simulink model "multi_model_sim_with_switching"  (R2013b)
settings: Solver=ode45  StartTime=0.0  StopTime=20  RelTol=1e-3
values from neighbouring files (symbols this model uses):
  C1d = [1 0]    [multi_model_sim_init.m]
  C1n = [C.Kp C.Ki]    [multi_model_sim_init.m]
  C2d = [1 0]    [multi_model_sim_init.m]
  C2n = [C.Kp C.Ki]    [multi_model_sim_init.m]
  C3d = [1 0]    [multi_model_sim_init.m]
  C3n = [C.Kp C.Ki]    [multi_model_sim_init.m]
  error_gain = 2    [multi_model_sim_init.m]
  P1d = [0.9125 1]    [multi_model_sim_init.m]
  P1n = [3.7]    [multi_model_sim_init.m]
  P2d = [1.075 1]    [multi_model_sim_init.m]
  P2n = [4]    [multi_model_sim_init.m]
  P3d = [0.7875 1]    [multi_model_sim_init.m]
  P3n = [1.78]    [multi_model_sim_init.m]
  Pd = [0.9 1]    [multi_model_sim_init.m]
  Pd_2 = [1 1]    [multi_model_sim_init.m]
  Pn = [1.8]    [multi_model_sim_init.m]
  Pn_2 = [4.2]    [multi_model_sim_init.m]
settings Model: Creator=alex  LastModifiedBy=alex

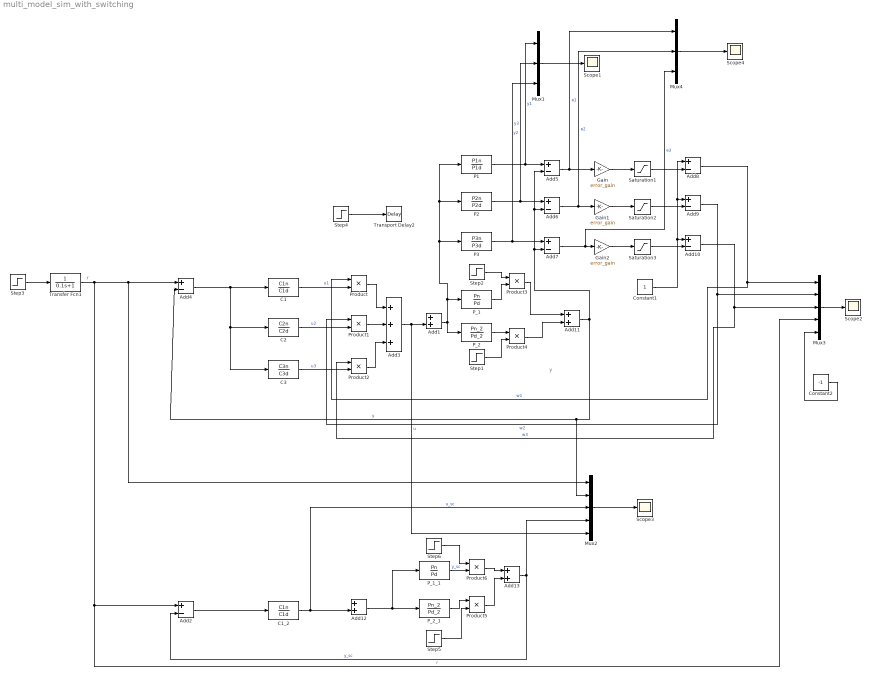
== system multi_model_sim_with_switching ==
  note: r
  note: y
  Add{1,11..13} (4 alike) : Sum
  Add{2,4..10} (8 alike) : Sum  Inputs=+-
  Add3 : Sum  Inputs=+++
  C1 : TransferFcn  Numerator=C1n  Denominator=C1d
  "C1_2 " : TransferFcn  Numerator=C1n  Denominator=C1d
  C2 : TransferFcn  Numerator=C2n  Denominator=C2d
  C3 : TransferFcn  Numerator=C3n  Denominator=C3d
  Constant1 : Constant
  Constant2 : Constant  Value=-1
  Gain : Gain  Gain=error_gain
  Gain1 : Gain  Gain=error_gain
  Gain2 : Gain  Gain=error_gain
  Mux1 : Mux  Inputs=3
  Mux2 : Mux  Inputs=5
  Mux3 : Mux  Inputs=5
  Mux4 : Mux  Inputs=3
  P1 : TransferFcn  Numerator=P1n  Denominator=P1d
  P2 : TransferFcn  Numerator=P2n  Denominator=P2d
  P3 : TransferFcn  Numerator=P3n  Denominator=P3d
  P_1 : TransferFcn  Numerator=Pn  Denominator=Pd
  P_1_1 : TransferFcn  Numerator=Pn  Denominator=Pd
  "P_2 " : TransferFcn  Numerator=Pn_2  Denominator=Pd_2
  "P_2_1 " : TransferFcn  Numerator=Pn_2  Denominator=Pd_2
  Product{,1..6} (7 alike) : Product
  Saturation1 : Saturate  UpperLimit=1  LowerLimit=0
  Saturation2 : Saturate  UpperLimit=1  LowerLimit=0
  Saturation3 : Saturate  UpperLimit=1  LowerLimit=0
  Scope{1..4} (4 alike) : Scope
      Scope1 settings: ShowLegends=on
      Scope2 settings: ShowLegends=on
      Scope3 settings: ShowLegends=on  SaveName=ScopeData3
      Scope4 settings: ShowLegends=on  SaveName=ScopeData2
  Step1 : Step  Time=5  Before=1  After=0  SampleTime=0
  Step2 : Step  Time=5  SampleTime=0
  Step3 : Step  SampleTime=0
  Step4 : Step  After=0.1  SampleTime=0
  Step5 : Step  Time=5  Before=1  After=0  SampleTime=0
  Step6 : Step  Time=5  SampleTime=0
  Transfer Fcn1 : TransferFcn  Denominator=[0.1 1]
  Transport Delay2 : TransportDelay  DelayTime=10
  wires:
  Mux2/1 -> Scope3/1
  Step3/1 -> Transfer Fcn1/1
  C1/1 -> Product/2  "u1"
  C2/1 -> Product1/2  "u2"
  C3/1 -> Product2/2  "u3"
  Product/1 -> Add3/1
  Product1/1 -> Add3/2
  Product2/1 -> Add3/3
  Add4/1 -> C1/1, C3/1, C2/1
  Transfer Fcn1/1 -> Mux2/1, Add4/1, Mux3/4, Add2/1  "r"
  P1/1 -> Mux1/1, Add5/1  "y1"
  P2/1 -> Add6/1, Mux1/2  "y2"
  P3/1 -> Add7/1, Mux1/3  "y3"
  Add5/1 -> Mux4/1, Gain/1  "e1"
  Add6/1 -> Mux4/2, Gain1/1  "e2"
  Add7/1 -> Mux4/3, Gain2/1  "e3"
  Gain/1 -> Saturation1/1
  Gain1/1 -> Saturation2/1
  Gain2/1 -> Saturation3/1
  Saturation1/1 -> Add8/2
  Saturation2/1 -> Add9/2
  Saturation3/1 -> Add10/2
  Step4/1 -> Transport Delay2/1
  Add11/1 -> Add4/2, Mux2/2, Add5/2, Add6/2, Add7/2  "y"
  Add9/1 -> Product1/1, Mux3/2  "w2"
  Add10/1 -> Mux3/3, Product2/1  "w3"
  Mux1/1 -> Scope1/1
  Add8/1 -> Mux3/1, Product/1  "w1"
  Mux3/1 -> Scope2/1
  Constant1/1 -> Add8/1, Add9/1, Add10/1
  Mux4/1 -> Scope4/1
  Add1/1 -> "P_2 "/1, P1/1, P2/1, P3/1, P_1/1
  Add3/1 -> Mux2/5, Add1/2  "u"
  Add2/1 -> "C1_2 "/1
  "C1_2 "/1 -> Mux2/3, Add12/2  "u_sc"
  Add12/1 -> "P_2_1 "/1, P_1_1/1
  Product4/1 -> Add11/2
  Step2/1 -> Product3/1
  P_1/1 -> Product3/2
  Product3/1 -> Add11/1
  "P_2 "/1 -> Product4/1
  Step1/1 -> Product4/2
  Product6/1 -> Add13/1
  Product5/1 -> Add13/2
  Step6/1 -> Product6/1
  P_1_1/1 -> Product6/2  "y_sc"
  "P_2_1 "/1 -> Product5/1
  Step5/1 -> Product5/2
  Add13/1 -> Add2/2, Mux2/4  "y_sc"
  Constant2/1 -> Mux3/5
